simulink model "trigo_tmp"  (Simulink 8.3)
settings: Solver=FixedStepDiscrete  StartTime=0.0  StopTime=10000.0  RelTol=1e-3
settings Model: Creator=scaife  LastModifiedBy=hbourbou  CovSFcnEnable=on  ExtModeAutoUpdateStatusClock=off
settings DataIOCC: SignalLoggingName=sigsOut
settings DebuggingCC: SaveWithParameterizedLinksMsg=none  SignalResolutionControl=TryResolveAllWithWarning  SolverPrmCheckMsg=none  MultiTaskDSMMsg=warning  MultiTaskCondExecSysMsg=none  FrameProcessingCompatibilityMsg=error  StateNameClashWarn=none
settings HardwareCC: TargetUnknown=on
settings SFSimCC: SimParseCustomCode=off

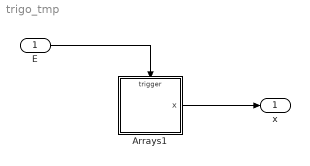
== system trigo_tmp ==
  E : Inport
  Arrays1 : Stateflow chart  TreatAsAtomicUnit=on
      settings: PermitHierarchicalResolution=ParametersOnly
  x : Outport
  wires:
  E/1 -> Arrays1/Trigger
  Arrays1/1(x) -> x/1

== stateflow chart Arrays1 ==
  state A/
    en:x=cos(1.0*x);
  state B/
    en:x=cos(10.0*x);
  state C/
    en:x=cos(2.0*x);
  (default) -> A
  C -> A : E
  A -> B : E
  B -> C : E
  data: x output int32 [0..100] =1.0
  events: E input RISING_EDGE_EVENT
